simulink model "projeto"  (R2015a)
settings: Solver=ode45  StartTime=0.0  StopTime=4.8  RelTol=1e-3
undefined symbols (not defined in the file): fa1, spf1
libraries: dsparch4 x12, dspvision x2, dspsrcs4 x2
settings Model: Creator=aluno  LastModifiedBy=aluno

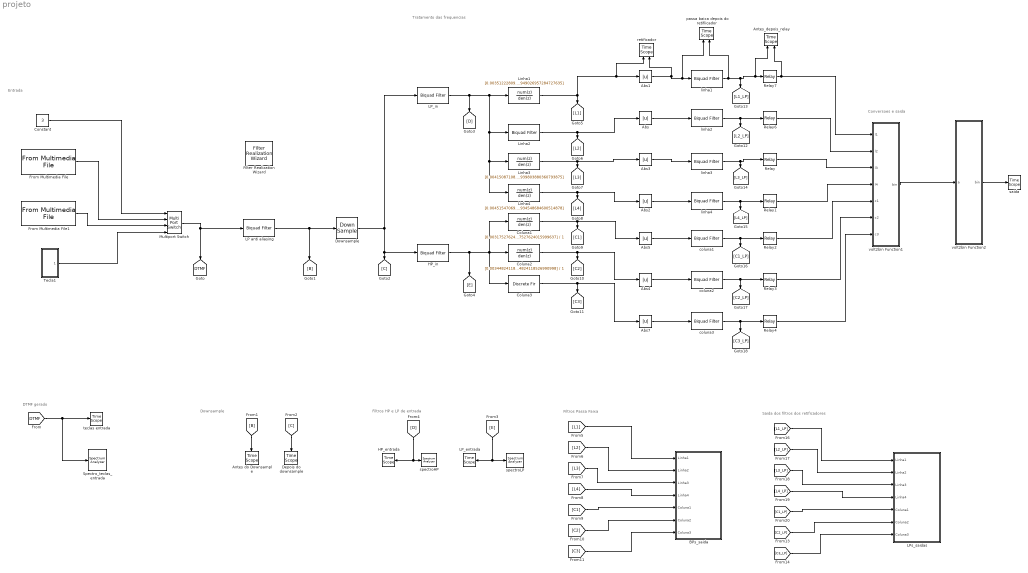
== system projeto ==
  note: Conversoes e saida
  note: Tratamento das frequencias
  note: Saida dos filtros dos retificadores
  note: Filtros Passa Faixa
  note: Filtros HP e LP de entrada
  note: DTMF gerado
  note: Downsample
  note: Entrada
  Abs{,1..5,7} (7 alike) : Abs
  Antes do Downsample : TimeScope  DefaultConfigurationName=spbscopes.TimeScopeBlockCfg
  Antes_depois_relay : TimeScope  DefaultConfigurationName=spbscopes.TimeScopeBlockCfg  NumInputPorts=2
  BPs_saida : Subsystem
  Coluna1 : DiscreteFilter  Tag=BlockMethodSubSystem  Numerator=[0.00317527624015999637 -0.00631791964356960556 0.00146396163617924292 0.00771826279994884245 -0.00934051380218392166 -0.00109136234220403856 0.0120341405745365126 -0.00923465058556301004 -0.00476203786087789002 0.0127156309640561998 -0.00552781432354629808 -0.00588002601387160612 0.00712097092971304517 -0.000876229832172920921 2.98345888493962144e-05 -0.00427463934333983941 -0.000569847441611774229 0.0153984016650217069 -0.0168920503385986132 -0.00995258662274600518 0.0381530793915716079 -0.0235188862821233274 -0.0309729272534876553 0.061436746169649413 -0.0178621283040634599 -0.0599494890707076566 0.0761792882426042539 0.00166667842380065971 -0.0882141515631010703 0.0754425958197448288 0.0302291926652146006 -0.105697383475048007 0.0581879997912456912 0.0581879997912456912 -0.105697383475048007 0.0302291926652146006 0.0754425958197448288 -0.0882141515631010703 0.00166667842380065971 0.0761792882426042539 -0.0599494890707076566 -0.0178621283040634599 0.061436746169649413 -0.0309729272534876553 -0.0235188862821233274 0.0381530793915716079 -0.00995258662274600518 -0.0168920503385986132 0.0153984016650217069 -0.000569847441611774229 -0.00427463934333983941 2.98345888493962144e-05 -0.000876229832172920921 0.00712097092971304517 -0.00588002601387160612 -0.00552781432354629808 0.0127156309640561998 -0.00476203786087789002 -0.00923465058556301004 0.0120341405745365126 -0.00109136234220403856 -0.00934051380218392166 0.00771826279994884245 0.00146396163617924292 -0.00631791964356960556 0.00317527624015999637]  Denominator=1  InputProcessing=Columns as channels (frame based)  a0EqualsOne=on
  Coluna2 : DiscreteFilter  Tag=BlockMethodSubSystem  Numerator=[0.00344824118526990998 0.00126039888081090276 -0.00527602717190759664 0.00558434647045385688 -0.00203437728666433114 -0.00250647536982737248 0.0045931372793634748 -0.00315077770308126465 0.000245352418174255916 0.00111057809355470986 -8.69266377316805616e-05 -0.00102662899348658111 -0.000700982249850059104 0.00512461819536735863 -0.00794691860279742035 0.00417355356245641129 0.00635984665855932486 -0.0166498800157385725 0.0167862094454364202 -0.00255404888816981824 -0.0186888091916770881 0.0311247443888415555 -0.0220266116709756758 -0.00656180261241871583 0.036184380649590217 -0.0437956273527211754 0.0195797490975324409 0.0229923136778496899 -0.0542772733591472267 0.0493862661953561391 -0.0079533861528964505 -0.0429901297955262648 0.0669546836251600497 -0.0446466379556028567 -0.0104950865118565752 0.0604345554301621013 -0.0694229754852827424 0.0301854813909569857 0.0301854813909569857 -0.0694229754852827424 0.0604345554301621013 -0.0104950865118565752 -0.0446466379556028567 0.0669546836251600497 -0.0429901297955262648 -0.0079533861528964505 0.0493862661953561391 -0.0542772733591472267 0.0229923136778496899 0.0195797490975324409 -0.0437956273527211754 0.036184380649590217 -0.00656180261241871583 -0.0220266116709756758 0.0311247443888415555 -0.0186888091916770881 -0.00255404888816981824 0.0167862094454364202 -0.0166498800157385725 0.00635984665855932486 0.00417355356245641129 -0.00794691860279742035 0.00512461819536735863 -0.000700982249850059104 -0.00102662899348658111 -8.69266377316805616e-05 0.00111057809355470986 0.000245352418174255916 -0.00315077770308126465 0.0045931372793634748 -0.00250647536982737248 -0.00203437728666433114 0.00558434647045385688 -0.00527602717190759664 0.00126039888081090276 0.00344824118526990998]  Denominator=1  InputProcessing=Columns as channels (frame based)  a0EqualsOne=on
  Coluna3 : DiscreteFir  Tag=BlockMethodSubSystem  Coefficients=[0.00512858771736026016 -0.00440011468462905321 0.00206810616070436616 0.000584402054986504316 -0.00212439799957778782 0.00185845678758979576 -0.000363398492304024769 -0.000740992991203455573 -0.000231308021719600187 0.0037894967901835018 -0.00850323253899488464 0.0113230861365750425 -0.00904966142145268923 0.000335273793437856731 0.0128498068952954993 -0.0252746644511767544 0.0303584373216764271 -0.0232995157212744566 0.00400048862667663676 0.0217881618600423502 -0.0440257528844798032 0.0523246359062617405 -0.0407142922500928345 0.0110392976172646179 0.0268045269015207248 -0.058275562161208147 0.0700347287349596254 -0.0557862216726810953 0.0194731452113693047 0.0257712970787470838 -0.0626764830671281553 0.0768373590084849706 -0.0626764830671281553 0.0257712970787470838 0.0194731452113693047 -0.0557862216726810953 0.0700347287349596254 -0.058275562161208147 0.0268045269015207248 0.0110392976172646179 -0.0407142922500928345 0.0523246359062617405 -0.0440257528844798032 0.0217881618600423502 0.00400048862667663676 -0.0232995157212744566 0.0303584373216764271 -0.0252746644511767544 0.0128498068952954993 0.000335273793437856731 -0.00904966142145268923 0.0113230861365750425 -0.00850323253899488464 0.0037894967901835018 -0.000231308021719600187 -0.000740992991203455573 -0.000363398492304024769 0.00185845678758979576 -0.00212439799957778782 0.000584402054986504316 0.00206810616070436616 -0.00440011468462905321 0.00512858771736026016]  InputProcessing=Columns as channels (frame based)
  Constant : Constant  Value=3
  Depois do downsample : TimeScope  DefaultConfigurationName=spbscopes.TimeScopeBlockCfg
  Downsample : DownSample  N=12  RateOptions=Allow multirate processing
  Filter Realization Wizard : dsparch4/Filter Realization Wizard
  From Multimedia File : dspvision/From Multimedia File  inputFilename=/home/aluno/Downloads/DTMF_teste.mp3  loop=on  numPlays=inf  outputStreams=Audio only  videoDataType=single  audioDataType=double  inheritSampleTime=on  userDefinedSampleTime=1/30  noAudioOutput=off  isIntensityVideo=off  fourcc=RGB  colorVideoFormat=Separate color signals  outputEOF=off  dataOrg=Column-major  audioFrameSize=spf1  computeAudioFrameSize=off  outSamplingMode=Sample based
  From Multimedia File1 : dspvision/From Multimedia File  inputFilename=/home/aluno/Downloads/DTMF_PROJ.mp3  loop=on  numPlays=inf  outputStreams=Audio only  videoDataType=single  audioDataType=double  inheritSampleTime=on  userDefinedSampleTime=1/30  noAudioOutput=off  isIntensityVideo=off  fourcc=RGB  colorVideoFormat=Separate color signals  outputEOF=off  dataOrg=Column-major  audioFrameSize=spf1  computeAudioFrameSize=off  outSamplingMode=Sample based
  HP_entrada : TimeScope  DefaultConfigurationName=spbscopes.TimeScopeBlockCfg
  HP_in : dsparch4/Biquad Filter  Tag=BlockMethodSubSystem  IIRFiltStruct=Direct form II  CoeffSource=Specify via dialog  BiQuadCoeffs=[1 -2 1 1 0.548806122620157932 0.842375048565931706;1 -2 1 1 1.229521681303404 0.556606553091564815]  a0Flag=Warning  IC=0  ICnum=0  ICden=0  InputProcessing=Columns as channels (frame based)  denAccumFracLength=30  denProdOutputFracLength=30  secondMemoryFracLength=15  roundingMode=Floor  overflowMode=off  ScaleValues=[0.323392231486443471;0.0817712179470402312;0.707945784384137911]  optimizeScaleValues=on  ScaleValueMode=Specify via input port (g)  scaleValueFracLength=14  FilterSource=Specify via dialog  FilterObject=Hm_biquad
  LP anti aliasing : dsparch4/Biquad Filter  Tag=BlockMethodSubSystem  IIRFiltStruct=Direct form II  CoeffSource=Specify via dialog  BiQuadCoeffs=[1 2 1 1 -1.63299316185545207 0.690598923241496965]  a0Flag=Warning  IC=0  ICnum=0  ICden=0  InputProcessing=Columns as channels (frame based)  denAccumFracLength=30  denProdOutputFracLength=30  secondMemoryFracLength=15  roundingMode=Floor  overflowMode=off  ScaleValues=[0.0144014403465112135;1]  optimizeScaleValues=on  ScaleValueMode=Specify via input port (g)  scaleValueFracLength=14  FilterSource=Specify via dialog  FilterObject=Hm_biquad
  LP_entrada : TimeScope  DefaultConfigurationName=spbscopes.TimeScopeBlockCfg
  LP_in : dsparch4/Biquad Filter  Tag=BlockMethodSubSystem  IIRFiltStruct=Direct form II  CoeffSource=Specify via dialog  BiQuadCoeffs=[1 2 1 1 0.37217462315301697 0.838626341666124153;1 2 1 1 -0.724064376464905735 0.428208293368322446]  a0Flag=Warning  IC=0  ICnum=0  ICden=0  InputProcessing=Columns as channels (frame based)  denAccumFracLength=30  denProdOutputFracLength=30  secondMemoryFracLength=15  roundingMode=Floor  overflowMode=off  ScaleValues=[0.552700241204785225;0.176035979225854178;0.707945784384137911]  optimizeScaleValues=on  ScaleValueMode=Specify via input port (g)  scaleValueFracLength=14  FilterSource=Specify via dialog  FilterObject=Hm_biquad
  LPs_saidas : Subsystem
  Linha1 : DiscreteFilter  Tag=BlockMethodSubSystem  Numerator=[0.00351222809187591578 -0.00518965103231234463 0.00540320400391500026 -1.22710095249474232e-20 -0.00540320400391500026 0.00518965103231234463 -0.00351222809187591578]  Denominator=[1 -2.20129354866606874 4.56179260782454055 -4.72039028124742988 4.48294603242865541 -2.12583611122697169 0.949026957284727635]  InputProcessing=Columns as channels (frame based)  a0EqualsOne=on
  Linha2 : dsparch4/Biquad Filter  Tag=BlockMethodSubSystem  IIRFiltStruct=Direct form II  CoeffSource=Specify via dialog  BiQuadCoeffs=[1 -0.599662804163566321 1 1 -0.546255897538132862 0.987883198896356896;1 -0.404393710721396626 1 1 -0.453649091452459796 0.987731587656940579;1 0 -1 1 -0.495289929065748036 0.968136236669282502]  a0Flag=Warning  IC=0  ICnum=0  ICden=0  InputProcessing=Columns as channels (frame based)  denAccumFracLength=30  denProdOutputFracLength=30  secondMemoryFracLength=15  roundingMode=Floor  overflowMode=off  ScaleValues=[0.408964239970837473;0.408964239970837473;0.0228015665474943091;1]  optimizeScaleValues=on  ScaleValueMode=Specify via input port (g)  scaleValueFracLength=14  FilterSource=Specify via dialog  FilterObject=Hm_biquad
  Linha3 : DiscreteFilter  Tag=BlockMethodSubSystem  Numerator=[0.00415087108653114292 -0.0018856135745880416 0.00431543366847822029 -5.29117758748448473e-21 -0.00431543366847822029 0.0018856135745880416 -0.00415087108653114292]  Denominator=[1 -0.676180608898375946 3.08843261455593954 -1.335545516480382 3.02521385731626058 -0.648763819705251321 0.939803880360793875]  InputProcessing=Columns as channels (frame based)  a0EqualsOne=on
  Linha4 : DiscreteFilter  Tag=BlockMethodSubSystem  Numerator=[0.00451547069762936286 0.000684717859183802606 0.00447659290202570472 2.09500291824054267e-21 -0.00447659290202570472 -0.000684717859183802606 -0.00451547069762936286]  Denominator=[1 0.22561564189167152 2.94699729245615227 0.441361927072614846 2.88129705362354205 0.215659855905080244 0.934548684600514878]  InputProcessing=Columns as channels (frame based)  a0EqualsOne=on
  Multiport Switch : MultiPortSwitch
  Relay{,1..4,6..7} (7 alike) : Relay  OnSwitchValue=0.15  OffSwitchValue=0.05
  Spectro_teclas_entrada : SpectrumAnalyzer
  Tecla1 : Subsystem  mask{linha=770, coluna=1336, spf1=spf1, fa1=fa1}
      mask prompts: linha "Frequencia da linha"; coluna "Frequencia da coluna"; spf1 "amostras por quadro"; fa1 "frequencia de amostragem"
  coluna1 : dsparch4/Biquad Filter  Tag=BlockMethodSubSystem  IIRFiltStruct=Direct form II  CoeffSource=Specify via dialog  BiQuadCoeffs=[1 2 1 1 -1.92266378299111951 0.92554489622593239]  a0Flag=Warning  IC=0  ICnum=0  ICden=0  InputProcessing=Columns as channels (frame based)  denAccumFracLength=30  denProdOutputFracLength=30  secondMemoryFracLength=15  roundingMode=Floor  overflowMode=off  ScaleValues=[0.000720278308703240899;1]  optimizeScaleValues=on  ScaleValueMode=Specify via input port (g)  scaleValueFracLength=14  FilterSource=Specify via dialog  FilterObject=Hm_biquad
  coluna2 : dsparch4/Biquad Filter  Tag=BlockMethodSubSystem  IIRFiltStruct=Direct form II  CoeffSource=Specify via dialog  BiQuadCoeffs=[1 2 1 1 -1.92266378299111951 0.92554489622593239]  a0Flag=Warning  IC=0  ICnum=0  ICden=0  InputProcessing=Columns as channels (frame based)  denAccumFracLength=30  denProdOutputFracLength=30  secondMemoryFracLength=15  roundingMode=Floor  overflowMode=off  ScaleValues=[0.000720278308703240899;1]  optimizeScaleValues=on  ScaleValueMode=Specify via input port (g)  scaleValueFracLength=14  FilterSource=Specify via dialog  FilterObject=Hm_biquad
  coluna3 : dsparch4/Biquad Filter  Tag=BlockMethodSubSystem  IIRFiltStruct=Direct form II  CoeffSource=Specify via dialog  BiQuadCoeffs=[1 2 1 1 -1.92266378299111951 0.92554489622593239]  a0Flag=Warning  IC=0  ICnum=0  ICden=0  InputProcessing=Columns as channels (frame based)  denAccumFracLength=30  denProdOutputFracLength=30  secondMemoryFracLength=15  roundingMode=Floor  overflowMode=off  ScaleValues=[0.000720278308703240899;1]  optimizeScaleValues=on  ScaleValueMode=Specify via input port (g)  scaleValueFracLength=14  FilterSource=Specify via dialog  FilterObject=Hm_biquad
  linha{1..4} (4 alike) : dsparch4/Biquad Filter  Tag=BlockMethodSubSystem  IIRFiltStruct=Direct form II  CoeffSource=Specify via dialog  BiQuadCoeffs=[1 2 1 1 -1.92266378299111951 0.92554489622593239]  a0Flag=Warning  IC=0  ICnum=0  ICden=0  InputProcessing=Columns as channels (frame based)  denAccumFracLength=30  denProdOutputFracLength=30  secondMemoryFracLength=15  roundingMode=Floor  overflowMode=off  ScaleValues=[0.000720278308703240899;1]  optimizeScaleValues=on  ScaleValueMode=Specify via input port (g)  scaleValueFracLength=14  FilterSource=Specify via dialog  FilterObject=Hm_biquad
  passa baixa depois do retifiicador : TimeScope  DefaultConfigurationName=spbscopes.TimeScopeBlockCfg  NumInputPorts=2
  "retificador " : TimeScope  DefaultConfigurationName=spbscopes.TimeScopeBlockCfg  NumInputPorts=2
  saida : TimeScope  DefaultConfigurationName=spbscopes.TimeScopeBlockCfg
  spectroHP : SpectrumAnalyzer
  spectroLP : SpectrumAnalyzer
  teclas entrada : TimeScope  DefaultConfigurationName=spbscopes.TimeScopeBlockCfg
  volt2bin Function1 : MATLAB Function  TreatAsAtomicUnit=on
  volt2bin Function2 : MATLAB Function  TreatAsAtomicUnit=on
  tag scope: DTMF=global
  wires:
  LP anti aliasing/1 -> Downsample/1, [B]
  [DTMF] -> Spectro_teclas_entrada/1, teclas entrada/1
  Tecla1/1(DTMF) -> Multiport Switch/4
  From Multimedia File1/1 -> Multiport Switch/3
  From Multimedia File/1 -> Multiport Switch/2
  Constant/1 -> Multiport Switch/1
  Multiport Switch/1 -> [DTMF], LP anti aliasing/1
  Downsample/1 -> HP_in/1, [C], LP_in/1
  HP_in/1 -> [E], Coluna3/1, Coluna1/1, Coluna2/1
  LP_in/1 -> [D], Linha2/1, Linha3/1, Linha4/1, Linha1/1
  Linha1/1 -> [L1], Abs1/1, "retificador "/1
  Linha2/1 -> [L2], Abs/1
  Linha3/1 -> [L3], Abs3/1
  Linha4/1 -> [L4], Abs2/1
  Coluna1/1 -> [C1], Abs5/1
  Coluna2/1 -> [C2], Abs4/1
  Coluna3/1 -> [C3], Abs7/1
  volt2bin Function1/1(bin) -> volt2bin Function2/1(a)
  Relay7/1 -> volt2bin Function1/1(l1), Antes_depois_relay/2
  Relay6/1 -> volt2bin Function1/2(l2)
  Relay/1 -> volt2bin Function1/3(l3)
  Relay1/1 -> volt2bin Function1/4(l4)
  Relay2/1 -> volt2bin Function1/5(c1)
  Relay3/1 -> volt2bin Function1/6(c2)
  Relay4/1 -> volt2bin Function1/7(c3)
  Abs1/1 -> "retificador "/2, passa baixa depois do retifiicador/1, linha1/1
  linha1/1 -> [L1_LP], Antes_depois_relay/1, Relay7/1, passa baixa depois do retifiicador/2
  linha2/1 -> [L2_LP], Relay6/1
  Abs/1 -> linha2/1
  Abs3/1 -> linha3/1
  linha3/1 -> [L3_LP], Relay/1
  linha4/1 -> [L4_LP], Relay1/1
  Abs2/1 -> linha4/1
  Abs5/1 -> coluna1/1
  coluna1/1 -> [C1_LP], Relay2/1
  coluna2/1 -> [C2_LP], Relay3/1
  Abs4/1 -> coluna2/1
  Abs7/1 -> coluna3/1
  coluna3/1 -> [C3_LP], Relay4/1
  [B] -> Antes do Downsample/1
  [C] -> Depois do downsample/1
  [E] -> LP_entrada/1, spectroLP/1
  [L1] -> BPs_saida/1(Linha1)
  [L2] -> BPs_saida/2(Linha2)
  [L3] -> BPs_saida/3(Linha3)
  [L4] -> BPs_saida/4(Linha4)
  [C1] -> BPs_saida/5(Coluna1)
  [C2] -> BPs_saida/6(Coluna2)
  [C3] -> BPs_saida/7(Coluna3)
  [L1_LP] -> LPs_saidas/1(Linha1)
  [L2_LP] -> LPs_saidas/2(Linha2)
  [C3_LP] -> LPs_saidas/7(Coluna3)
  [C2_LP] -> LPs_saidas/6(Coluna2)
  [C1_LP] -> LPs_saidas/5(Coluna1)
  [L4_LP] -> LPs_saidas/4(Linha4)
  [L3_LP] -> LPs_saidas/3(Linha3)
  volt2bin Function2/1(bin) -> saida/1
  [D] -> spectroHP/1, HP_entrada/1

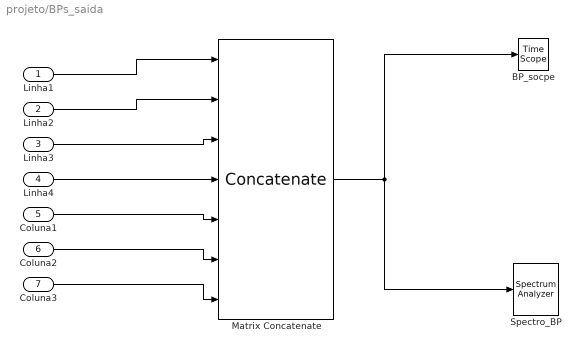
== system projeto/BPs_saida ==
  Linha1 : Inport
  Linha2 : Inport  Port=2
  Linha3 : Inport  Port=3
  Linha4 : Inport  Port=4
  Coluna1 : Inport  Port=5
  Coluna2 : Inport  Port=6
  Coluna3 : Inport  Port=7
  BP_socpe : TimeScope  DefaultConfigurationName=spbscopes.TimeScopeBlockCfg
  Matrix Concatenate : Concatenate  NumInputs=7  Mode=Multidimensional array  ConcatenateDimension=2
  Spectro_BP : SpectrumAnalyzer
  wires:
  Matrix Concatenate/1 -> BP_socpe/1, Spectro_BP/1
  Linha3/1 -> Matrix Concatenate/3
  Linha4/1 -> Matrix Concatenate/4
  Coluna2/1 -> Matrix Concatenate/6
  Coluna3/1 -> Matrix Concatenate/7
  Linha2/1 -> Matrix Concatenate/2
  Linha1/1 -> Matrix Concatenate/1
  Coluna1/1 -> Matrix Concatenate/5

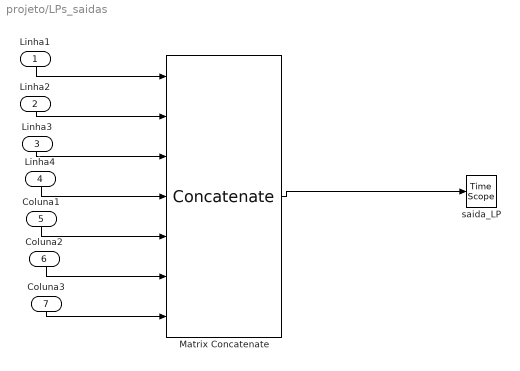
== system projeto/LPs_saidas ==
  Linha1 : Inport
  Linha2 : Inport  Port=2
  Linha3 : Inport  Port=3
  Linha4 : Inport  Port=4
  Coluna1 : Inport  Port=5
  Coluna2 : Inport  Port=6
  Coluna3 : Inport  Port=7
  Matrix Concatenate : Concatenate  NumInputs=7  Mode=Multidimensional array  ConcatenateDimension=2
  saida_LP : TimeScope  DefaultConfigurationName=spbscopes.TimeScopeBlockCfg
  wires:
  Linha3/1 -> Matrix Concatenate/3
  Coluna3/1 -> Matrix Concatenate/7
  Coluna2/1 -> Matrix Concatenate/6
  Coluna1/1 -> Matrix Concatenate/5
  Linha4/1 -> Matrix Concatenate/4
  Matrix Concatenate/1 -> saida_LP/1
  Linha1/1 -> Matrix Concatenate/1
  Linha2/1 -> Matrix Concatenate/2

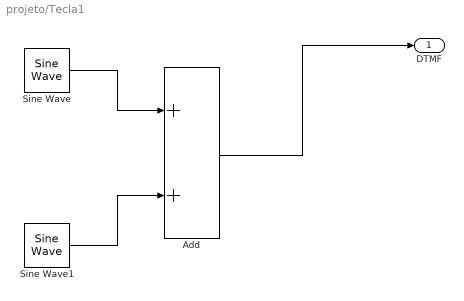
== system projeto/Tecla1 ==
  Add : Sum
  Sine Wave : dspsrcs4/Sine Wave  Amplitude=1  Frequency=coluna  Phase=0  SampleMode=Discrete  OutComplex=Real  CompMethod=Trigonometric fcn  TableSize=Speed  SampleTime=1/fa1  SamplesPerFrame=spf1  ResetState=Restart at time zero  dataType=double  wordLen=16  udDataType=sfix(16)  fracBitsMode=Best precision  numFracBits=15  OutDataTypeStr=double  LastOutDataTypeStr=double
  Sine Wave1 : dspsrcs4/Sine Wave  Amplitude=1  Frequency=linha  Phase=0  SampleMode=Discrete  OutComplex=Real  CompMethod=Trigonometric fcn  TableSize=Speed  SampleTime=1/fa1  SamplesPerFrame=spf1  ResetState=Restart at time zero  dataType=double  wordLen=16  udDataType=sfix(16)  fracBitsMode=Best precision  numFracBits=15  OutDataTypeStr=double  LastOutDataTypeStr=double
  DTMF : Outport
  wires:
  Sine Wave/1 -> Add/1
  Sine Wave1/1 -> Add/2
  Add/1 -> DTMF/1

== matlab function projeto/volt2bin Function2 ==
  data: a input; bin output
function bin = fcn(a)
bin = bi2de(a);
end

== matlab function projeto/volt2bin Function1 ==
  data: l1 input; l2 input; l3 input; l4 input; c1 input; bin output; c2 input; c3 input
function bin = fcn(l1,l2,l3,l4,c1,c2,c3)
spf1 = size(l1,1);
binario = zeros(spf1,4);

for k = 1:spf1

    %ERROS
    if ((l1(k,:) + l2(k,:) + l3(k,:) + l4(k,:)) > 1) || ((c1(k,:) + c2(k,:) + c3(k,:)) > 1)
        binario(k,:) = [0 1 1 1]; %14
    end;

    if ((l1(k,:) + l2(k,:) + l3(k,:) + l4(k,:) + c1(k,:) + c2(k,:) + c3(k,:)) == 1)
        binario(k,:) = [1 0 1 1]; %13
    end;

    %o da esquerda eh o LSB
    x = [l1(k,:) l2(k,:) l3(k,:) l4(k,:) c1(k,:) c2(k,:) c3(k,:)];
    convert_x = bi2de(x);
        switch convert_x
            case 0
                binario(k,:) = [0 0 0 0];
            case 40 % numero 0
                binario(k,:) = [0 1 0 1]; % 10

            case 17 % numero 1
                binario(k,:) = [1 0 0 0]; % 1

            case 33 % numero 2
                binario(k,:) = [0 1 0 0]; % 2

            case 65 % numero 3
                binario(k,:) = [1 1 0 0] ; % 3

            case 18 % numero 4
                binario(k,:) = [0 0 1 0]; % 4

            case 34 % numero 5
                binario(k,:) = [1 0 1 0]; % 5

            case 66 % numero 6
                binario(k,:) = [0 1 1 0]; % 6

            case 20 %numero 7
                binario(k,:) = [1 1 1 0]; % 7

            case 36 %numero 8
                binario(k,:) = [0 0 0 1]; % 8

            case 68 %numero 9
                binario(k,:) = [1 0 0 1]; % 9

            case 24 %numero *
                binario(k,:) = [0 0 1 1];  %12

            case 72 %numero #
                binario(k,:) = [1 1 1 1]; % 15
        end
        bin = binario;
end
end
